simulink model "Main_Sim_Kylle"  (R2018b)
settings: Solver=ode5  StartTime=0.0  StopTime=20000  FixedStep=simParams.sample_time_s  RelTol=1e-3  EnableMultiTasking=on
undefined symbols (not defined in the file or in its folder): DiscIntNeverNeededParam, FSW_Lib, fswParams, MEKF_lib, q_body, r_eci_km, satelliteDynamics_lib, simParams, v_eci_km, w_body_radps
libraries: vrlib x6, aerolibutil x5, CrossProdMatrix_lib x4, sharedutil x4, dspmathops x2, actuators_lib x1, CDH_command_lib x1, Environment_lib x1, MEKF_Conversion_lib x1, sharedtransform x1, actuator_processing_lib x1, allocation_lib x1
(part 1 of 2)
settings Model: Creator=devantormey  LastModifiedBy=kylle
settings OptimizationCC: LifeSpan=inf
settings DebuggingCC: SFUnexpectedBacktrackingDiag=warning  SFNoUnconditionalDefaultTransitionDiag=warning
settings SFSimCC: SimUseLocalCustomCode=off
settings RTWCC: RTWUseLocalCustomCode=off
settings CodeAppCC: StateflowObjectComments=on
settings GRTTargetCC: TargetLangStandard=C89/C90 (ANSI)  GeneratePreprocessorConditionals=Disable all
settings ConfigComp: CovMetricSettings=dw  CovHtmlReporting=on  CovSaveCumulativeToWorkspaceVar=on  CovSaveSingleToWorkspaceVar=on  CovExternalEMLEnable=off

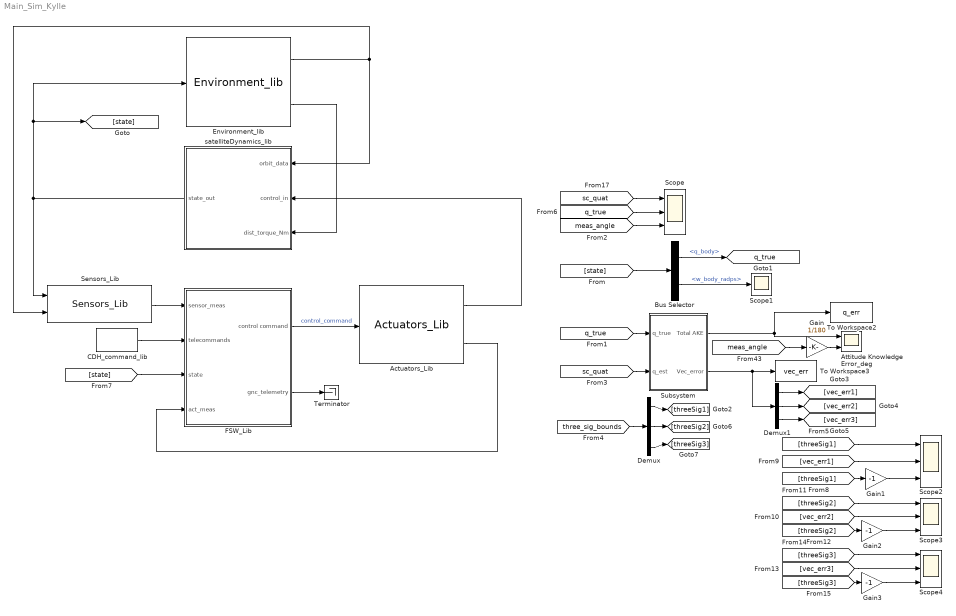
== system Main_Sim_Kylle ==
  Actuators_Lib : actuators_lib/Actuators_Lib  SystemSampleTime=-1
  "Attitude Knowledge Error_deg " : Scope  NumInputPorts=2
  Bus Selector : BusSelector  OutputSignals=q_body,w_body_radps
  CDH_command_lib : CDH_command_lib/CDH_command_lib  SystemSampleTime=-1
  Demux : Demux  Outputs=3
  Demux1 : Demux  Outputs=3
  Environment_lib : Environment_lib/Environment_lib  SystemSampleTime=-1
  FSW_Lib : Subsystem  AncestorBlock=FSW_Lib/FSW_Lib
  Gain : Gain  Gain=1/180
  Gain1 : Gain  Gain=-1
  Gain2 : Gain  Gain=-1
  Gain3 : Gain  Gain=-1
  Scope{,2..4} (4 alike) : Scope  NumInputPorts=3
  Scope1 : Scope
  Sensors_Lib : Sensors_Lib/Sensors_Lib  SystemSampleTime=-1
  Subsystem : Subsystem
  Terminator : Terminator
  To Workspace2 : ToWorkspace  VariableName=q_err  SaveFormat=Timeseries  SampleTime=-1
  To Workspace3 : ToWorkspace  VariableName=vec_err  SaveFormat=Timeseries  SampleTime=-1
  satelliteDynamics_lib : Subsystem  AncestorBlock=satelliteDynamics_lib/satelliteDynamics_lib
  tag scope: q_true=global
  wires:
  FSW_Lib/2(gnc_telemetry) -> Terminator/1
  CDH_command_lib/1 -> FSW_Lib/2(telecommands)
  [state] -> Bus Selector/1
  Bus Selector/2 -> Scope1/1  "<w_body_radps>"
  Bus Selector/1 -> [q_true]  "<q_body>"
  Subsystem/1(Total AKE) -> To Workspace2/1, "Attitude Knowledge Error_deg "/1
  [sc_quat] -> Subsystem/2("q_est ")
  [q_true] -> Subsystem/1("q_true ")
  [q_true] -> Scope/2
  Actuators_Lib/1 -> satelliteDynamics_lib/2(control_in)
  Actuators_Lib/2 -> FSW_Lib/4(act_meas)
  Sensors_Lib/1 -> FSW_Lib/1(sensor_meas)
  FSW_Lib/1(control command) -> Actuators_Lib/1  "control_command"
  [sc_quat] -> Scope/1
  satelliteDynamics_lib/1(state_out) -> Sensors_Lib/1, [state], Environment_lib/1
  Environment_lib/1 -> Sensors_Lib/2, satelliteDynamics_lib/1(orbit_data)
  Environment_lib/2 -> satelliteDynamics_lib/3(dist_torque_Nm)
  [state] -> FSW_Lib/3(state)
  [meas_angle] -> Gain/1
  [meas_angle] -> Scope/3
  [three_sig_bounds] -> Demux/1
  Subsystem/2(Vec_error) -> Demux1/1, To Workspace3/1
  Gain1/1 -> Scope2/3
  Demux/1 -> [threeSig1]
  [threeSig1] -> Scope2/1
  [threeSig1] -> Gain1/1
  Demux1/1 -> [vec_err1]
  Demux1/3 -> [vec_err3]
  Demux1/2 -> [vec_err2]
  [vec_err1] -> Scope2/2
  [vec_err2] -> Scope3/2
  Demux/2 -> [threeSig2]
  Demux/3 -> [threeSig3]
  [threeSig2] -> Scope3/1
  Gain2/1 -> Scope3/3
  [threeSig2] -> Gain2/1
  [threeSig3] -> Scope4/1
  [vec_err3] -> Scope4/2
  [threeSig3] -> Gain3/1
  Gain3/1 -> Scope4/3
  Gain/1 -> "Attitude Knowledge Error_deg "/2

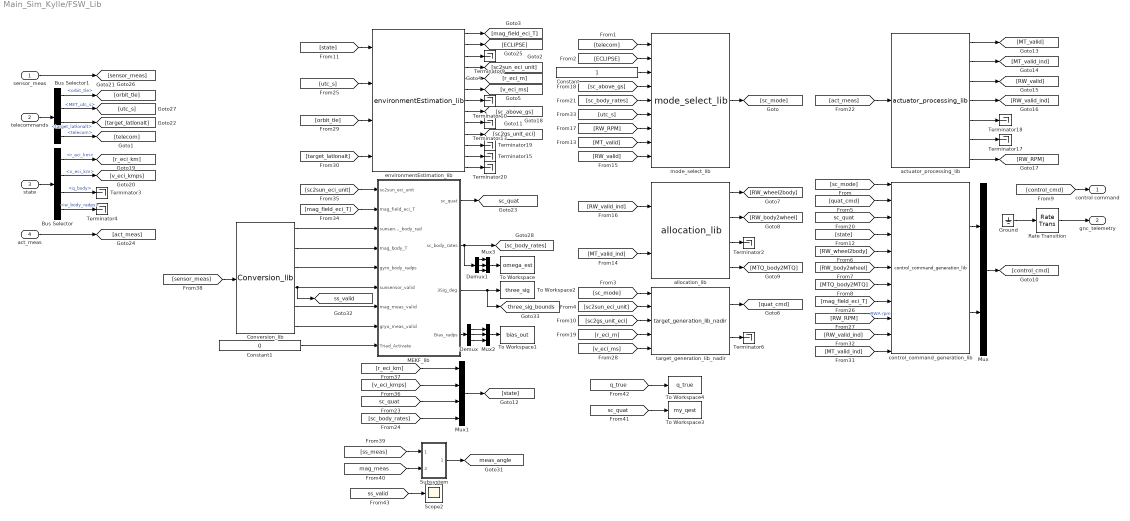
== system Main_Sim_Kylle/FSW_Lib ==
  sensor_meas : Inport
  telecommands : Inport  Port=2
  state : Inport  Port=3
  act_meas : Inport  Port=4
  Bus Selector : BusSelector  OutputSignals=r_eci_km,v_eci_km,q_body,w_body_radps
  Bus Selector1 : BusSelector  OutputSignals=orbit_tle,MET_utc_s,target_latlonalt,telecom
  Constant : Constant
  Constant1 : Constant  Value=0
  Conversion_lib : MEKF_Conversion_lib/Conversion_lib  SystemSampleTime=-1
  Demux : Demux  Outputs=3
  Demux1 : Demux  Outputs=3
  Ground : Ground
  MEKF_lib : Subsystem  AncestorBlock=MEKF_lib/MEKF_lib  TreatAsAtomicUnit=on
      settings: RTWFcnNameOpts=Use subsystem name  RTWFileNameOpts=Use subsystem name
  Mux : Mux  Inputs=[4 5]
  Mux1 : Mux  Inputs=[3 3 4 3]
  Mux2 : Mux  Inputs=3
  Mux3 : Mux  Inputs=3
  Rate Transition : RateTransition  OutPortSampleTime=fswParams.sample_time_s
  Scope2 : Scope
  Subsystem : Subsystem
  Terminator{2..4,6,9..10,13,15,17..20} (12 alike) : Terminator
  To Workspace : ToWorkspace  VariableName=omega_est  SaveFormat=Timeseries  SampleTime=-1
  To Workspace1 : ToWorkspace  VariableName=bias_out  SaveFormat=Timeseries  SampleTime=-1
  To Workspace2 : ToWorkspace  VariableName=three_sig  SaveFormat=Timeseries  SampleTime=-1
  To Workspace3 : ToWorkspace  VariableName=my_qest  SaveFormat=Timeseries  SampleTime=-1
  To Workspace4 : ToWorkspace  VariableName=q_true  SaveFormat=Timeseries  SampleTime=-1
  actuator_processing_lib : actuator_processing_lib/actuator_processing_lib  SystemSampleTime=-1
  allocation_lib : allocation_lib/allocation_lib  SystemSampleTime=-1
  control_command_generation_lib : control_command_generation_lib/control_command_generation_lib  SystemSampleTime=-1
  environmentEstimation_lib : evironmentEstimation_lib/environmentEstimation_lib  SystemSampleTime=-1
  mode_select_lib : mode_select_lib/mode_select_lib  SystemSampleTime=-1
  target_generation_lib_nadir : target_gen_lib_nadir/target_generation_lib_nadir  SystemSampleTime=-1
  control command : Outport
  gnc_telemetry : Outport  Port=2
  tag scope: meas_angle=global, sc_quat=global, ss_valid=global, three_sig_bounds=global
  wires:
  Bus Selector1/4 -> [telecom]  "<telecom>"
  [r_eci_m] -> target_generation_lib_nadir/4
  [utc_s] -> mode_select_lib/6
  [MT_valid_ind] -> control_command_generation_lib/11
  [RW_valid_ind] -> control_command_generation_lib/10
  Rate Transition/1 -> gnc_telemetry/1
  target_generation_lib_nadir/1 -> [quat_cmd]
  [target_latlonalt] -> environmentEstimation_lib/4
  Bus Selector1/3 -> [target_latlonalt]  "<target_latlonalt>"
  Bus Selector1/1 -> [orbit_tle]  "<orbit_tle>"
  [v_eci_ms] -> target_generation_lib_nadir/5
  [RW_RPM] -> control_command_generation_lib/9  "RWA rpm"
  [mag_field_eci_T] -> control_command_generation_lib/8
  Bus Selector1/2 -> [utc_s]  "<MET_utc_s>"
  environmentEstimation_lib/11 -> Terminator19/1
  environmentEstimation_lib/13 -> Terminator20/1
  environmentEstimation_lib/12 -> Terminator15/1
  [act_meas] -> actuator_processing_lib/1
  actuator_processing_lib/7 -> [RW_RPM]
  actuator_processing_lib/6 -> Terminator17/1
  actuator_processing_lib/5 -> Terminator18/1
  actuator_processing_lib/4 -> [RW_valid_ind]
  actuator_processing_lib/3 -> [RW_valid]
  actuator_processing_lib/2 -> [MT_valid_ind]
  actuator_processing_lib/1 -> [MT_valid]
  act_meas/1 -> [act_meas]
  [state] -> control_command_generation_lib/4
  [state] -> environmentEstimation_lib/1
  state/1 -> Bus Selector/1
  [sc2gs_unit_eci] -> target_generation_lib_nadir/3
  [orbit_tle] -> environmentEstimation_lib/3
  [utc_s] -> environmentEstimation_lib/2
  environmentEstimation_lib/10 -> [sc2gs_unit_eci]
  environmentEstimation_lib/9 -> Terminator13/1
  environmentEstimation_lib/8 -> [sc_above_gs]
  environmentEstimation_lib/7 -> Terminator10/1
  environmentEstimation_lib/6 -> [v_eci_ms]
  environmentEstimation_lib/5 -> [r_eci_m]
  environmentEstimation_lib/4 -> [sc2sun_eci_unit]
  environmentEstimation_lib/3 -> Terminator9/1
  environmentEstimation_lib/2 -> [ECLIPSE]
  environmentEstimation_lib/1 -> [mag_field_eci_T]
  Mux/1 -> [control_cmd]
  control_command_generation_lib/1 -> Mux/1
  control_command_generation_lib/2 -> Mux/2
  [MTQ_body2MTQ] -> control_command_generation_lib/7
  [RW_body2wheel] -> control_command_generation_lib/6
  allocation_lib/4 -> [MTQ_body2MTQ]
  allocation_lib/3 -> Terminator2/1
  [RW_wheel2body] -> control_command_generation_lib/5
  allocation_lib/2 -> [RW_body2wheel]
  allocation_lib/1 -> [RW_wheel2body]
  [sc_quat] -> control_command_generation_lib/3
  [MT_valid_ind] -> allocation_lib/2
  [RW_valid_ind] -> allocation_lib/1
  [quat_cmd] -> control_command_generation_lib/2
  target_generation_lib_nadir/2 -> Terminator6/1
  [sc2sun_eci_unit] -> target_generation_lib_nadir/2
  [sc_mode] -> target_generation_lib_nadir/1
  [RW_valid] -> mode_select_lib/9
  [MT_valid] -> mode_select_lib/8
  Constant/1 -> mode_select_lib/3
  [RW_RPM] -> mode_select_lib/7
  [sc_body_rates] -> mode_select_lib/5
  [sc_above_gs] -> mode_select_lib/4
  [ECLIPSE] -> mode_select_lib/2
  [telecom] -> mode_select_lib/1
  [sc_mode] -> control_command_generation_lib/1
  mode_select_lib/1 -> [sc_mode]
  [control_cmd] -> control command/1
  Ground/1 -> Rate Transition/1
  telecommands/1 -> Bus Selector1/1
  [sc_quat] -> Mux1/3
  [sc_body_rates] -> Mux1/4
  Mux1/1 -> [state]
  Conversion_lib/5 -> MEKF_lib/7(mag_meas_valid)
  Conversion_lib/4 -> MEKF_lib/6(sunsensor_valid), [ss_valid]
  Conversion_lib/3 -> MEKF_lib/5(gyro_body_radps)
  Conversion_lib/2 -> MEKF_lib/4(mag_body_T)
  Conversion_lib/1 -> MEKF_lib/3(sunsensor_body_rad)
  [sc2sun_eci_unit] -> MEKF_lib/1(sc2sun_eci_unit)
  [mag_field_eci_T] -> MEKF_lib/2(mag_field_eci_T)
  Bus Selector/1 -> [r_eci_km]  "<r_eci_km>"
  Bus Selector/2 -> [v_eci_kmps]  "<v_eci_km>"
  [r_eci_km] -> Mux1/1
  [v_eci_kmps] -> Mux1/2
  Bus Selector/3 -> Terminator3/1  "<q_body>"
  Bus Selector/4 -> Terminator4/1  "<w_body_radps>"
  sensor_meas/1 -> [sensor_meas]
  [sensor_meas] -> Conversion_lib/1
  MEKF_lib/1(sc_quat) -> [sc_quat]
  MEKF_lib/2(sc_body_rates) -> Demux1/1, [sc_body_rates]
  [ss_meas] -> Subsystem/1(In1)
  [mag_meas] -> Subsystem/2(In2)
  Subsystem/1(Out1) -> [meas_angle]
  [q_true] -> To Workspace4/1
  MEKF_lib/4(Bias_radps) -> Demux/1
  Mux2/1 -> To Workspace1/1
  Demux/1 -> Mux2/1
  Demux/2 -> Mux2/2
  Demux/3 -> Mux2/3
  Demux1/1 -> Mux3/1
  Demux1/2 -> Mux3/2
  Demux1/3 -> Mux3/3
  Mux3/1 -> To Workspace/1
  MEKF_lib/3("3Sig_deg ") -> [three_sig_bounds], To Workspace2/1
  Constant1/1 -> MEKF_lib/9(Triad_Activate)
  Conversion_lib/6 -> MEKF_lib/8(gryo_meas_valid)
  [ss_valid] -> Scope2/1
  [sc_quat] -> To Workspace3/1

== system Main_Sim_Kylle/Subsystem ==
  "q_true " : Inport
  "q_est " : Inport  Port=2
  Acos : Trigonometry  Operator=acos
  Demux3 : Demux
  Gain1 : Gain  Gain=180/pi
  Gain6 : Gain  Gain=180/pi*2
  Mux : Mux  Inputs=3
  Quaternion Conjugate : aerolibutil/Quaternion Conjugate
      settings: SourceProductName=Aerospace Blockset  SourceProductBaseCode=AE
  Quaternion Multiplication : aerolibutil/Quaternion Multiplication
  Total AKE : Outport
  Vec_error : Outport  Port=2
  wires:
  "q_true "/1 -> Quaternion Conjugate/1
  Acos/1 -> Gain6/1
  Mux/1 -> Gain1/1
  Gain6/1 -> Total AKE/1
  Demux3/2 -> Mux/1
  Quaternion Conjugate/1 -> Quaternion Multiplication/1
  Demux3/1 -> Acos/1
  Demux3/3 -> Mux/2
  "q_est "/1 -> Quaternion Multiplication/2
  Demux3/4 -> Mux/3
  Gain1/1 -> Vec_error/1
  Quaternion Multiplication/1 -> Demux3/1

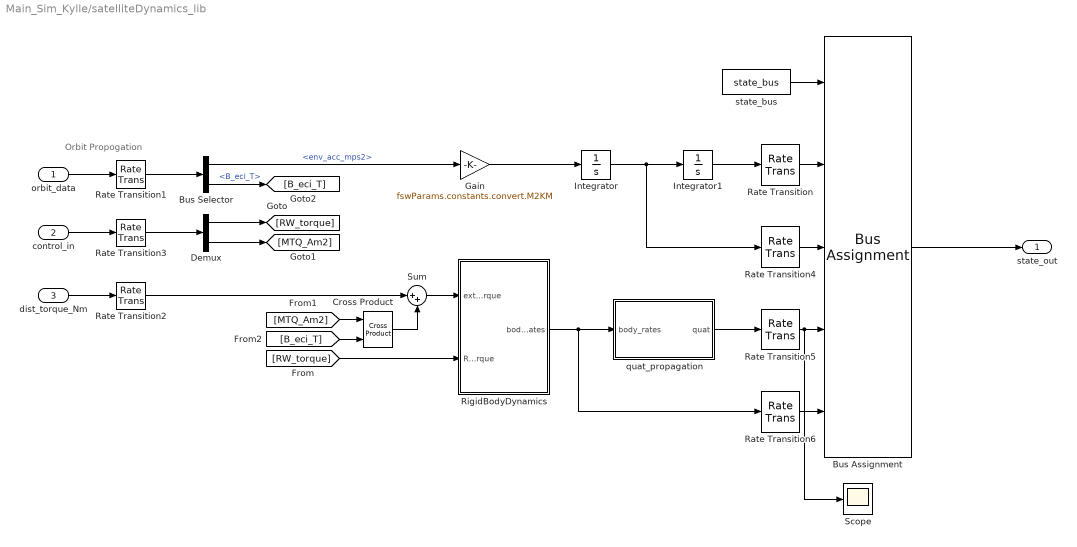
== system Main_Sim_Kylle/satelliteDynamics_lib ==
  note: Orbit Propogation
  orbit_data : Inport
  control_in : Inport  Port=2
  dist_torque_Nm : Inport  Port=3
  Bus Assignment : BusAssignment  AssignedSignals=r_eci_km,v_eci_km,q_body,w_body_radps
  Bus Selector : BusSelector  OutputSignals=env_acc_mps2,B_eci_T
  Cross Product : vrlib/Utilities/Cross Product
      settings: SourceProductBaseCode=VR
  Demux : Demux  Outputs=[3 3]
  Gain : Gain  Gain=fswParams.constants.convert.M2KM
  Integrator : Integrator  InitialCondition=simParams.initialConditions.v0
  Integrator1 : Integrator  InitialCondition=simParams.initialConditions.r0
  Rate Transition : RateTransition  InitialCondition=simParams.initialConditions.r0
  Rate Transition1 : RateTransition  OutPortSampleTime=simParams.sample_time_s
  Rate Transition2 : RateTransition  OutPortSampleTime=simParams.sample_time_s
  Rate Transition3 : RateTransition  OutPortSampleTime=simParams.sample_time_s
  Rate Transition4 : RateTransition  InitialCondition=simParams.initialConditions.v0
  Rate Transition5 : RateTransition  InitialCondition=simParams.initialConditions.q0
  Rate Transition6 : RateTransition  InitialCondition=simParams.initialConditions.w0
  RigidBodyDynamics : Subsystem
  Scope : Scope
  Sum : Sum  Inputs=|++
  quat_propagation : Subsystem
  state_bus : state_bus/state_bus  SystemSampleTime=-1
  state_out : Outport
  wires:
  Rate Transition6/1 -> Bus Assignment/5
  Rate Transition5/1 -> Scope/1, Bus Assignment/4
  Rate Transition4/1 -> Bus Assignment/3
  Rate Transition/1 -> Bus Assignment/2
  state_bus/1 -> Bus Assignment/1
  Sum/1 -> RigidBodyDynamics/1(external_torque)
  [MTQ_Am2] -> Cross Product/1
  [RW_torque] -> RigidBodyDynamics/2(RW_torque)
  Demux/2 -> [MTQ_Am2]
  Demux/1 -> [RW_torque]
  Rate Transition3/1 -> Demux/1
  Rate Transition2/1 -> Sum/1
  RigidBodyDynamics/1(body_rates) -> quat_propagation/1(body_rates), Rate Transition6/1
  quat_propagation/1(quat) -> Rate Transition5/1
  dist_torque_Nm/1 -> Rate Transition2/1
  Bus Assignment/1 -> state_out/1
  Gain/1 -> Integrator/1
  Integrator1/1 -> Rate Transition/1
  Integrator/1 -> Integrator1/1, Rate Transition4/1
  control_in/1 -> Rate Transition3/1
  orbit_data/1 -> Rate Transition1/1
  Bus Selector/1 -> Gain/1  "<env_acc_mps2>"
  Rate Transition1/1 -> Bus Selector/1
  Bus Selector/2 -> [B_eci_T]  "<B_eci_T>"
  [B_eci_T] -> Cross Product/2
  Cross Product/1 -> Sum/2

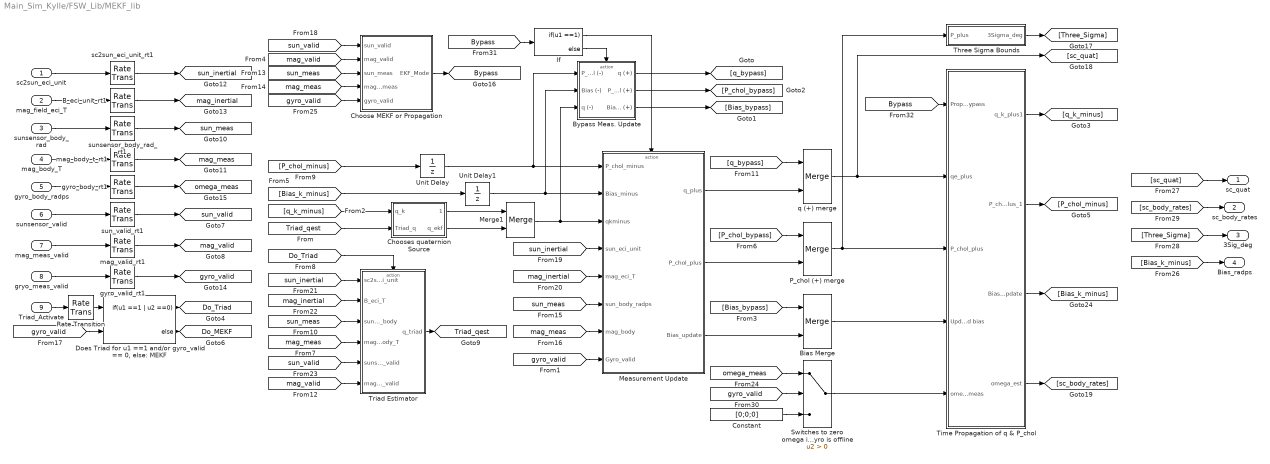
== system Main_Sim_Kylle/FSW_Lib/MEKF_lib ==
  sc2sun_eci_unit : Inport
  mag_field_eci_T : Inport  Port=2
  sunsensor_body_rad : Inport  Port=3
  mag_body_T : Inport  Port=4
  gyro_body_radps : Inport  Port=5
  sunsensor_valid : Inport  Port=6
  mag_meas_valid : Inport  Port=7
  gryo_meas_valid : Inport  Port=8
  Triad_Activate : Inport  Port=9
  B_eci_unit_rt1 : RateTransition  InitialCondition=fswParams.estimation.ic.B_eci_unit_rt  OutPortSampleTime=fswParams.sample_time_s
  Bias Merge : Merge
  Bypass Meas. Update : Subsystem  TreatAsAtomicUnit=on
  Choose MEKF or Propagation : Subsystem
  Chooses quaternion Source : Subsystem
  Constant : Constant  Value=[0;0;0]
  "Does Triad for u1 ==1 and/or gyro_valid == 0, else: MEKF" : If  NumInputs=2  IfExpression=u1 ==1 | u2 ==0
  If : If  IfExpression=u1 ==1
  Measurement Update : Subsystem  TreatAsAtomicUnit=on
  Merge1 : Merge
  P_chol (+) merge : Merge
  Rate Transition : RateTransition  OutPortSampleTime=fswParams.sample_time_s
  "Switches to zero omega if Gyro is offline " : Switch  Criteria=u2 > Threshold
  Three Sigma Bounds : Subsystem
  Time Propagation of q & P_chol : Subsystem
  Triad Estimator : Subsystem  TreatAsAtomicUnit=on
  Unit Delay : UnitDelay  InitialCondition=fswParams.estimation.ic.Pchol_init  SampleTime=fswParams.sample_time_s
  Unit Delay1 : UnitDelay  InitialCondition=fswParams.estimation.ic.Beta_init  SampleTime=fswParams.sample_time_s
  gyro_body_rt1 : RateTransition  InitialCondition=fswParams.estimation.ic.gyro_meas_rt  OutPortSampleTime=fswParams.sample_time_s
  gyro_valid_rt1 : RateTransition  InitialCondition=fswParams.estimation.ic.gyro_valid_rt  OutPortSampleTime=fswParams.sample_time_s
  mag_body_t_rt1 : RateTransition  InitialCondition=fswParams.estimation.ic.mag_body_rt  OutPortSampleTime=fswParams.sample_time_s
  mag_valid_rt1 : RateTransition  InitialCondition=fswParams.estimation.ic.mag_valid_rt  OutPortSampleTime=fswParams.sample_time_s
  q (+) merge : Merge
  sc2sun_eci_unit_rt1 : RateTransition  InitialCondition=fswParams.estimation.ic.sc2sun_eci_unit_rt  OutPortSampleTime=fswParams.sample_time_s
  sun_valid_rt1 : RateTransition  InitialCondition=fswParams.estimation.ic.sun_valid_rt  OutPortSampleTime=fswParams.sample_time_s
  sunsensor_body_rad_rt1 : RateTransition  InitialCondition=fswParams.estimation.ic.sunsensor_body_rad_rt  OutPortSampleTime=fswParams.sample_time_s
  sc_quat : Outport
  sc_body_rates : Outport  Port=2
  "3Sig_deg " : Outport  Port=3
  Bias_radps : Outport  Port=4
  tag scope: Bypass=global, Do_MEKF=global, Do_Triad=global, Triad_qest=global, gyro_valid=global, mag_inertial=global, mag_meas=global, mag_valid=global, omega_meas=global, sun_inertial=global, sun_meas=global, sun_valid=global
  wires:
  [gyro_valid] -> "Switches to zero omega if Gyro is offline "/2
  [Bypass] -> If/1
  [Bypass] -> Time Propagation of q & P_chol/1("Prop_bypass ")
  Bias Merge/1 -> Time Propagation of q & P_chol/4(Updated bias)
  "Switches to zero omega if Gyro is offline "/1 -> Time Propagation of q & P_chol/5(omega_meas)
  [sc_body_rates] -> sc_body_rates/1
  Time Propagation of q & P_chol/4(omega_est) -> [sc_body_rates]
  [Three_Sigma] -> "3Sig_deg "/1
  Three Sigma Bounds/1(3Sigma_deg) -> [Three_Sigma]
  [sc_quat] -> sc_quat/1
  [Bias_k_minus] -> Bias_radps/1
  [gyro_valid] -> Choose MEKF or Propagation/5(gyro_valid)
  [gyro_valid] -> "Does Triad for u1 ==1 and/or gyro_valid == 0, else: MEKF"/2
  [mag_inertial] -> Triad Estimator/2(B_eci_T)
  [mag_valid] -> Triad Estimator/6(magsensor_valid)
  [sun_inertial] -> Triad Estimator/1(sc2sun_eci_unit)
  [mag_meas] -> Triad Estimator/4(mag_meas_body_T)
  [sun_valid] -> Triad Estimator/5(sunsensor_valid)
  [Do_Triad] -> Triad Estimator/Action
  [sun_meas] -> Triad Estimator/3(sun_meas_rad_body)
  [mag_meas] -> Choose MEKF or Propagation/4(mag_meas)
  [sun_meas] -> Choose MEKF or Propagation/3(sun_meas)
  [mag_valid] -> Choose MEKF or Propagation/2(mag_valid)
  [sun_valid] -> Choose MEKF or Propagation/1(sun_valid)
  [gyro_valid] -> Measurement Update/8(Gyro_valid)
  [Triad_qest] -> Chooses quaternion Source/2(Triad_q)
  Chooses quaternion Source/2(q_ekf) -> Merge1/2
  Chooses quaternion Source/1(Triad_qest) -> Merge1/1
  [q_k_minus] -> Chooses quaternion Source/1(q_k)
  Triad Estimator/1(q_triad) -> [Triad_qest]
  [sun_inertial] -> Measurement Update/4(sun_eci_unit)
  [mag_inertial] -> Measurement Update/5("mag_eci_T ")
  [omega_meas] -> "Switches to zero omega if Gyro is offline "/1
  gyro_body_rt1/1 -> [omega_meas]
  gyro_valid_rt1/1 -> [gyro_valid]
  B_eci_unit_rt1/1 -> [mag_inertial]
  sc2sun_eci_unit_rt1/1 -> [sun_inertial]
  Choose MEKF or Propagation/1(EKF_Mode) -> [Bypass]
  Merge1/1 -> Measurement Update/3(qkminus), Bypass Meas. Update/3(q (-))
  Unit Delay1/1 -> Bypass Meas. Update/2(Bias (-)), Measurement Update/2(Bias_minus)
  Unit Delay/1 -> Bypass Meas. Update/1(P_chol (-)), Measurement Update/1(P_chol_minus)
  mag_valid_rt1/1 -> [mag_valid]
  sun_valid_rt1/1 -> [sun_valid]
  [mag_meas] -> Measurement Update/7(mag_body)
  mag_body_t_rt1/1 -> [mag_meas]
  sunsensor_body_rad_rt1/1 -> [sun_meas]
  [sun_meas] -> Measurement Update/6(sun_body_radps)
  gyro_body_radps/1 -> gyro_body_rt1/1
  mag_meas_valid/1 -> mag_valid_rt1/1
  sunsensor_valid/1 -> sun_valid_rt1/1
  "Does Triad for u1 ==1 and/or gyro_valid == 0, else: MEKF"/2 -> [Do_MEKF]
  "Does Triad for u1 ==1 and/or gyro_valid == 0, else: MEKF"/1 -> [Do_Triad]
  Triad_Activate/1 -> Rate Transition/1
  Rate Transition/1 -> "Does Triad for u1 ==1 and/or gyro_valid == 0, else: MEKF"/1
  sunsensor_body_rad/1 -> sunsensor_body_rad_rt1/1
  mag_body_T/1 -> mag_body_t_rt1/1
  mag_field_eci_T/1 -> B_eci_unit_rt1/1
  sc2sun_eci_unit/1 -> sc2sun_eci_unit_rt1/1
  Time Propagation of q & P_chol/1(q_k_plus1) -> [q_k_minus]
  Time Propagation of q & P_chol/2(P_chol_plus_1) -> [P_chol_minus]
  If/1 -> Measurement Update/Action
  If/2 -> Bypass Meas. Update/Action
  [Bias_k_minus] -> Unit Delay1/1
  [P_chol_minus] -> Unit Delay/1
  Measurement Update/1(q_plus) -> q (+) merge/2
  Measurement Update/3(Bias_update) -> Bias Merge/2
  Bypass Meas. Update/1(q (+)) -> [q_bypass]
  [q_bypass] -> q (+) merge/1
  [Bias_bypass] -> Bias Merge/1
  Bypass Meas. Update/2(P_chol (+)) -> [P_chol_bypass]
  Bypass Meas. Update/3(Bias (+)) -> [Bias_bypass]
  gryo_meas_valid/1 -> gyro_valid_rt1/1
  Constant/1 -> "Switches to zero omega if Gyro is offline "/3
  P_chol (+) merge/1 -> Time Propagation of q & P_chol/3(P_chol_plus), Three Sigma Bounds/1(P_plus)
  [P_chol_bypass] -> P_chol (+) merge/1
  Measurement Update/2(P_chol_plus) -> P_chol (+) merge/2
  Time Propagation of q & P_chol/3(Bias_Update) -> [Bias_k_minus]
  q (+) merge/1 -> [sc_quat], Time Propagation of q & P_chol/2(qe_plus)

== system Main_Sim_Kylle/FSW_Lib/Subsystem ==
  In1 : Inport
  In2 : Inport  Port=2
  Acos : Trigonometry  Operator=acos
  Divide : Product  Inputs=*/
  Dot Product : DotProduct  InputSameDT=on  OutDataTypeStr=Inherit: Inherit via internal rule
  Dot Product1 : DotProduct  InputSameDT=on  OutDataTypeStr=Inherit: Inherit via internal rule
  Dot Product2 : DotProduct  InputSameDT=on  OutDataTypeStr=Inherit: Inherit via internal rule
  Gain : Gain  Gain=180/pi
  Multiply : Product
  Sqrt : Sqrt  SaturateOnIntegerOverflow=on
  Sqrt1 : Sqrt  SaturateOnIntegerOverflow=on
  Out1 : Outport
  wires:
  In1/1 -> Dot Product1/2, Dot Product1/1, Dot Product/1
  Divide/1 -> Acos/1
  Dot Product2/1 -> Sqrt1/1
  In2/1 -> Dot Product2/2, Dot Product2/1, Dot Product/2
  Sqrt1/1 -> Multiply/2
  Sqrt/1 -> Multiply/1
  Dot Product/1 -> Divide/1
  Dot Product1/1 -> Sqrt/1
  Multiply/1 -> Divide/2
  Acos/1 -> Gain/1
  Gain/1 -> Out1/1

== system Main_Sim_Kylle/satelliteDynamics_lib/RigidBodyDynamics ==
  external_torque : Inport
  RW_torque : Inport  Port=2
  Discrete-Time Integrator : DiscreteIntegrator  InitialCondition=[0;0;0]  SampleTime=-1  ICPrevOutput=DiscIntNeverNeededParam  ICPrevScaledInput=DiscIntNeverNeededParam
  Integrator : Integrator  InitialCondition=simParams.initialConditions.w0
  dynamics : Subsystem
  body_rates : Outport
  wires:
  dynamics/1(omega_dot) -> Integrator/1
  external_torque/1 -> dynamics/1(external_torque_Nm)
  Integrator/1 -> dynamics/4(omega_radps), body_rates/1
  Discrete-Time Integrator/1 -> dynamics/3(rw_momentum_Nms)
  RW_torque/1 -> Discrete-Time Integrator/1, dynamics/2(rw_torque_Nm)

== system Main_Sim_Kylle/satelliteDynamics_lib/quat_propagation ==
  body_rates : Inport
  Gain1 : Gain  Gain=1/2
  Integrator : Integrator  InitialCondition=simParams.initialConditions.q0
  MATLAB Function : MATLAB Function  TreatAsAtomicUnit=on
  Product : Product  Multiplication=Matrix(*)  RndMeth=Zero
  Quaternion Normalize : sharedutil/Quaternion Normalize  aMode=aMode
      settings: SourceProductName=Aerospace Blockset  SourceProductBaseCode=AE
  quat : Outport
  wires:
  MATLAB Function/1(Omega) -> Gain1/1
  body_rates/1 -> MATLAB Function/1(w)
  Quaternion Normalize/1 -> Product/2, quat/1
  Gain1/1 -> Product/1
  Integrator/1 -> Quaternion Normalize/1
  Product/1 -> Integrator/1

== system Main_Sim_Kylle/FSW_Lib/MEKF_lib/Bypass Meas. Update ==
  P_chol (-) : Inport
  Bias (-) : Inport  Port=2
  q (-) : Inport  Port=3
  Action Port : ActionPort  ActionType=else
  q (+) : Outport
  P_chol (+) : Outport  Port=2
  Bias (+) : Outport  Port=3
  wires:
  P_chol (-)/1 -> P_chol (+)/1
  Bias (-)/1 -> Bias (+)/1
  q (-)/1 -> q (+)/1

== system Main_Sim_Kylle/FSW_Lib/MEKF_lib/Choose MEKF or Propagation ==
  sun_valid : Inport
  mag_valid : Inport  Port=2
  sun_meas : Inport  Port=3
  mag_meas : Inport  Port=4
  gyro_valid : Inport  Port=5
  AND : Logic  Inputs=4  AllPortsSameDT=off  OutDataTypeStr=boolean
  Decides if Angle Between Measurements < 2.5 deg : Subsystem  AncestorBlock=MEKF_lib/MEKF_lib/Triad_alg/Triad/Angle_between_vectors
  EKF_Mode : Outport
  wires:
  gyro_valid/1 -> AND/4
  mag_meas/1 -> Decides if Angle Between Measurements < 2.5 deg/2(mag_meas_T_body)
  sun_meas/1 -> Decides if Angle Between Measurements < 2.5 deg/1(sun_meas_rad_body)
  mag_valid/1 -> AND/2
  sun_valid/1 -> AND/1
  AND/1 -> EKF_Mode/1
  Decides if Angle Between Measurements < 2.5 deg/1(Parallel_Protection) -> AND/3

== system Main_Sim_Kylle/FSW_Lib/MEKF_lib/Chooses quaternion Source ==
  q_k : Inport
  Triad_q : Inport  Port=2
  If Action Subsystem2 : Subsystem  TreatAsAtomicUnit=on
  Unit Delay2 : UnitDelay  InitialCondition=fswParams.estimation.ic.quat_est_init  SampleTime=fswParams.sample_time_s
  Triad_qest : Outport
  q_ekf : Outport  Port=2
  wires:
  Triad_q/1 -> Triad_qest/1
  If Action Subsystem2/1(Out1) -> q_ekf/1
  q_k/1 -> Unit Delay2/1
  [Do_MEKF] -> If Action Subsystem2/Action
  Unit Delay2/1 -> If Action Subsystem2/1(In1)

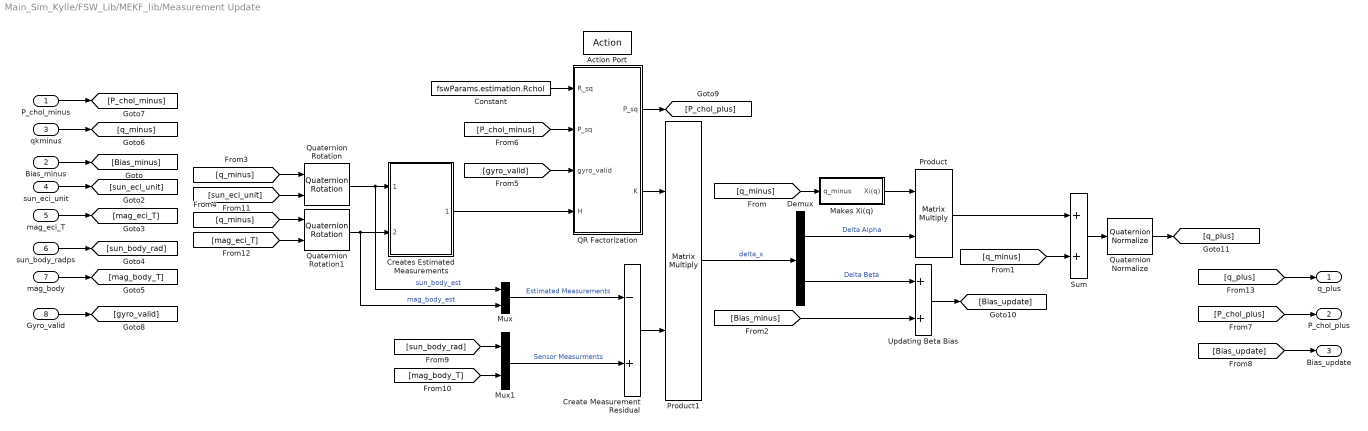
== system Main_Sim_Kylle/FSW_Lib/MEKF_lib/Measurement Update ==
  P_chol_minus : Inport
  Bias_minus : Inport  Port=2
  qkminus : Inport  Port=3
  sun_eci_unit : Inport  Port=4
  "mag_eci_T " : Inport  Port=5
  sun_body_radps : Inport  Port=6
  mag_body : Inport  Port=7
  Gyro_valid : Inport  Port=8
  Action Port : ActionPort  ActionType=then
  Constant : Constant  Value=fswParams.estimation.Rchol  VectorParams1D=off
  Create Measurement Residual : Sum  Inputs=-+
  Creates Estimated Measurements : Subsystem
  Demux : Demux  Outputs=2
  Makes Xi(q) : Subsystem
  Mux : Mux  Inputs=2
  Mux1 : Mux  Inputs=2
  Product : Product  Inputs=**  Multiplication=Matrix(*)
  Product1 : Product  Multiplication=Matrix(*)
  QR Factorization : MATLAB Function  TreatAsAtomicUnit=on
  Quaternion Normalize : sharedutil/Quaternion Normalize  aMode=aMode
      settings: SourceProductName=Aerospace Blockset  SourceProductBaseCode=AE
  Quaternion Rotation : aerolibutil/Quaternion Rotation
  Quaternion Rotation1 : aerolibutil/Quaternion Rotation
  Sum : Sum
  "Updating Beta Bias " : Sum
  q_plus : Outport
  P_chol_plus : Outport  Port=2
  Bias_update : Outport  Port=3
  wires:
  [q_plus] -> q_plus/1
  Quaternion Normalize/1 -> [q_plus]
  [mag_eci_T] -> Quaternion Rotation1/2
  [sun_eci_unit] -> Quaternion Rotation/2
  [mag_body_T] -> Mux1/2
  [sun_body_rad] -> Mux1/1
  Gyro_valid/1 -> [gyro_valid]
  [Bias_update] -> Bias_update/1
  "Updating Beta Bias "/1 -> [Bias_update]
  [P_chol_plus] -> P_chol_plus/1
  QR Factorization/1(P_sq) -> [P_chol_plus]
  [P_chol_minus] -> QR Factorization/2("P_sq ")
  [gyro_valid] -> QR Factorization/3(gyro_valid)
  P_chol_minus/1 -> [P_chol_minus]
  mag_body/1 -> [mag_body_T]
  "mag_eci_T "/1 -> [mag_eci_T]
  sun_eci_unit/1 -> [sun_eci_unit]
  sun_body_radps/1 -> [sun_body_rad]
  [q_minus] -> Quaternion Rotation1/1
  [q_minus] -> Quaternion Rotation/1
  [Bias_minus] -> "Updating Beta Bias "/2
  Bias_minus/1 -> [Bias_minus]
  Constant/1 -> QR Factorization/1(R_sq)
  QR Factorization/2(K) -> Product1/1
  Creates Estimated Measurements/1(H_matrix) -> QR Factorization/4(H)
  [q_minus] -> Makes Xi(q)/1(q_minus)
  qkminus/1 -> [q_minus]
  Quaternion Rotation/1 -> Creates Estimated Measurements/1(sun_body_hat), Mux/1  "sun_body_est"
  Quaternion Rotation1/1 -> Creates Estimated Measurements/2(mag_body_hat), Mux/2  "mag_body_est"
  Create Measurement Residual/1 -> Product1/2
  Makes Xi(q)/1(Xi(q)) -> Product/1
  Demux/1 -> Product/2  "Delta Alpha"
  Product1/1 -> Demux/1  "delta_x"
  Product/1 -> Sum/1
  Sum/1 -> Quaternion Normalize/1
  Mux/1 -> Create Measurement Residual/1  "Estimated Measurements"
  Demux/2 -> "Updating Beta Bias "/1  "Delta Beta"
  Mux1/1 -> Create Measurement Residual/2  "Sensor Measurments"
  [q_minus] -> Sum/2

== system Main_Sim_Kylle/FSW_Lib/MEKF_lib/Three Sigma Bounds ==
  P_plus : Inport
  Abs : Abs
  Demux : Demux  Outputs=2
  Extract Diagonal : S-Function  FunctionName=sdspdiag2  Parameters=mode  SFunctionDeploymentMode=off  EnableBusSupport=off  mask(Extract Diagonal){}
      mask help: Extract the main diagonal of a full matrix.
      mask init:
      | mode = 2;
      | x = [.58 .87 NaN 0.12 0.45 0.45 0.12 0.12 NaN 0.525 0.525 0.475 0.475 0.525 0.525 0.565 0.525 ];
      | y = [ 0.8 0.2 NaN 0.2 0.2 0.8 0.8 0.2 NaN 0.435 0.475 0.475 0.525 0.525 0.565 0.5 0.435 ];
      mask Help: eval('blocksethelp');
      mask Display:
      | plot(x,y);
      | port_label('input',1,'A');
      | port_label('output',1,'D');
  Multiply : Gain  Gain=3*180/pi
  Terminator : Terminator
  3Sigma_deg : Outport
  wires:
  Demux/2 -> Terminator/1
  Demux/1 -> Abs/1
  Extract Diagonal/1 -> Demux/1
  Abs/1 -> Multiply/1
  P_plus/1 -> Extract Diagonal/1
  Multiply/1 -> 3Sigma_deg/1

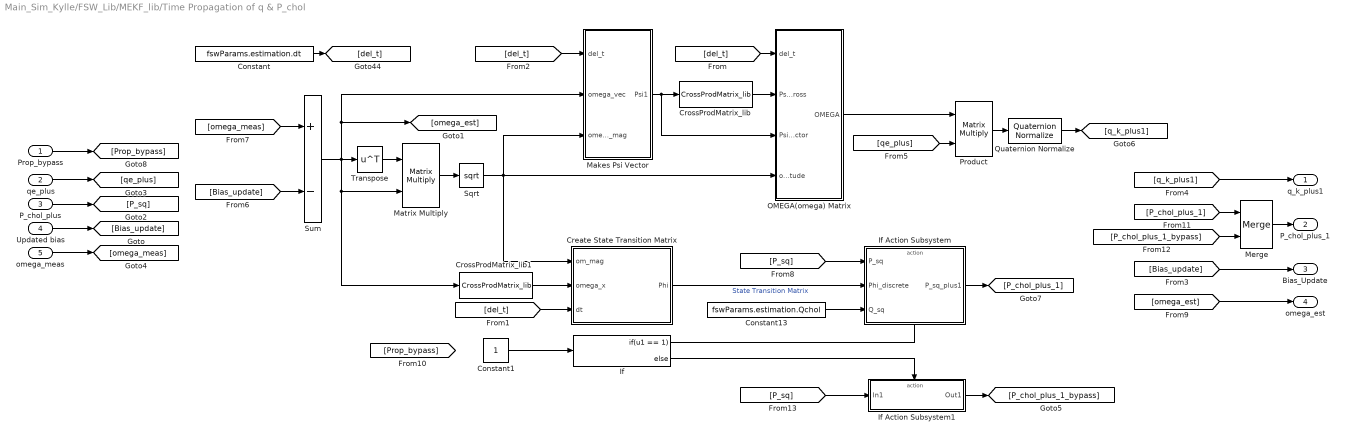
== system Main_Sim_Kylle/FSW_Lib/MEKF_lib/Time Propagation of q & P_chol ==
  "Prop_bypass " : Inport
  qe_plus : Inport  Port=2
  P_chol_plus : Inport  Port=3
  Updated bias : Inport  Port=4
  omega_meas : Inport  Port=5
  Constant : Constant  Value=fswParams.estimation.dt
  Constant1 : Constant
  Constant13 : Constant  Value=fswParams.estimation.Qchol  VectorParams1D=off
  Create State Transition Matrix : MATLAB Function  TreatAsAtomicUnit=on
  CrossProdMatrix_lib : CrossProdMatrix_lib/CrossProdMatrix_lib  SystemSampleTime=-1
  CrossProdMatrix_lib1 : CrossProdMatrix_lib/CrossProdMatrix_lib  SystemSampleTime=-1
  If : If  IfExpression=u1 == 1
  If Action Subsystem : Subsystem  TreatAsAtomicUnit=on
  If Action Subsystem1 : Subsystem  TreatAsAtomicUnit=on
  Makes Psi Vector : Subsystem
  Matrix Multiply : Product  Multiplication=Matrix(*)
  Merge : Merge
  OMEGA(omega) Matrix : Subsystem
  Product : Product  Multiplication=Matrix(*)
  Quaternion Normalize : sharedutil/Quaternion Normalize  aMode=aMode
      settings: SourceProductName=Aerospace Blockset  SourceProductBaseCode=AE
  Sqrt : Sqrt  SaturateOnIntegerOverflow=on
  Sum : Sum  Inputs=+-
  Transpose : Math  Operator=transpose  SaturateOnIntegerOverflow=on
  q_k_plus1 : Outport
  P_chol_plus_1 : Outport  Port=2
  Bias_Update : Outport  Port=3
  omega_est : Outport  Port=4
  wires:
  [P_sq] -> If Action Subsystem1/1(In1)
  "Prop_bypass "/1 -> [Prop_bypass]
  [P_chol_plus_1] -> Merge/1
  Merge/1 -> P_chol_plus_1/1
  [P_chol_plus_1_bypass] -> Merge/2
  If Action Subsystem1/1(Out1) -> [P_chol_plus_1_bypass]
  If/2 -> If Action Subsystem1/Action
  If/1 -> If Action Subsystem/Action
  If Action Subsystem/1(P_sq_plus1) -> [P_chol_plus_1]
  [q_k_plus1] -> q_k_plus1/1
  Quaternion Normalize/1 -> [q_k_plus1]
  [P_sq] -> If Action Subsystem/1("P_sq ")
  [omega_meas] -> Sum/1
  [Bias_update] -> Sum/2
  omega_meas/1 -> [omega_meas]
  P_chol_plus/1 -> [P_sq]
  Updated bias/1 -> [Bias_update]
  [qe_plus] -> Product/2
  qe_plus/1 -> [qe_plus]
  [omega_est] -> omega_est/1
  [Bias_update] -> Bias_Update/1
  Constant13/1 -> If Action Subsystem/3(Q_sq)
  Create State Transition Matrix/1(Phi) -> If Action Subsystem/2(Phi_discrete)  "State Transition Matrix"
  OMEGA(omega) Matrix/1(OMEGA) -> Product/1
  CrossProdMatrix_lib/1 -> OMEGA(omega) Matrix/2(Psi_cross)
  Makes Psi Vector/1(Psi1) -> OMEGA(omega) Matrix/3(Psi_vector), CrossProdMatrix_lib/1
  [del_t] -> OMEGA(omega) Matrix/1(del_t)
  CrossProdMatrix_lib1/1 -> Create State Transition Matrix/2(omega_x)
  Sqrt/1 -> Create State Transition Matrix/1(om_mag), Makes Psi Vector/3(omega_mag), OMEGA(omega) Matrix/4(omega_magnitude)
  Transpose/1 -> Matrix Multiply/1
  Matrix Multiply/1 -> Sqrt/1
  Constant/1 -> [del_t]
  Sum/1 -> Makes Psi Vector/2(omega_vec), [omega_est], CrossProdMatrix_lib1/1, Matrix Multiply/2, Transpose/1
  [del_t] -> Makes Psi Vector/1(del_t)
  [del_t] -> Create State Transition Matrix/3(dt)
  Product/1 -> Quaternion Normalize/1
  Constant1/1 -> If/1

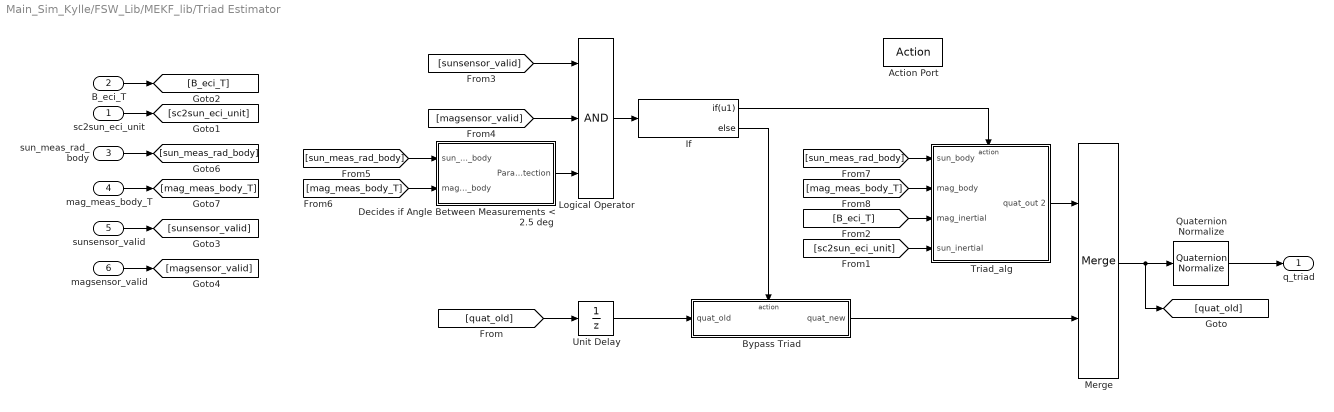
== system Main_Sim_Kylle/FSW_Lib/MEKF_lib/Triad Estimator ==
  sc2sun_eci_unit : Inport
  B_eci_T : Inport  Port=2
  sun_meas_rad_body : Inport  Port=3
  mag_meas_body_T : Inport  Port=4
  sunsensor_valid : Inport  Port=5
  magsensor_valid : Inport  Port=6
  Action Port : ActionPort  ActionType=then
  Bypass Triad : Subsystem  TreatAsAtomicUnit=on
  Decides if Angle Between Measurements < 2.5 deg : Subsystem
  If : If  IfExpression=u1
  Logical Operator : Logic  Inputs=3  AllPortsSameDT=off  OutDataTypeStr=boolean
  Merge : Merge
  Quaternion Normalize : sharedutil/Quaternion Normalize  aMode=aMode
      settings: SourceProductName=Aerospace Blockset  SourceProductBaseCode=AE
  Triad_alg : Subsystem  TreatAsAtomicUnit=on
  Unit Delay : UnitDelay  InitialCondition=fswParams.estimation.ic.quat_est_init  SampleTime=fswParams.sample_time_s
  q_triad : Outport
  wires:
  Quaternion Normalize/1 -> q_triad/1
  [B_eci_T] -> Triad_alg/3("mag_inertial ")
  [sc2sun_eci_unit] -> Triad_alg/4(sun_inertial)
  B_eci_T/1 -> [B_eci_T]
  sc2sun_eci_unit/1 -> [sc2sun_eci_unit]
  [mag_meas_body_T] -> Decides if Angle Between Measurements < 2.5 deg/2(mag_meas_T_body)
  mag_meas_body_T/1 -> [mag_meas_body_T]
  [sun_meas_rad_body] -> Decides if Angle Between Measurements < 2.5 deg/1(sun_meas_rad_body)
  sun_meas_rad_body/1 -> [sun_meas_rad_body]
  [magsensor_valid] -> Logical Operator/2
  magsensor_valid/1 -> [magsensor_valid]
  [sunsensor_valid] -> Logical Operator/1
  sunsensor_valid/1 -> [sunsensor_valid]
  [mag_meas_body_T] -> Triad_alg/2(mag_body)
  [sun_meas_rad_body] -> Triad_alg/1(sun_body)
  Decides if Angle Between Measurements < 2.5 deg/1(Parallel_Protection) -> Logical Operator/3
  Unit Delay/1 -> Bypass Triad/1(quat_old)
  [quat_old] -> Unit Delay/1
  Logical Operator/1 -> If/1
  Bypass Triad/1(quat_new) -> Merge/2
  Triad_alg/1(quat_out 2) -> Merge/1
  If/2 -> Bypass Triad/Action
  If/1 -> Triad_alg/Action
  Merge/1 -> [quat_old], Quaternion Normalize/1

== system Main_Sim_Kylle/satelliteDynamics_lib/RigidBodyDynamics/dynamics ==
  note: Euler's equation: J dw/dt = T_{ext} + T_{rw} - w x ( Jw + h_w )
      |
      | RW being momentum exchange devices do NOT create
      | an external torque on the s/c
  external_torque_Nm : Inport
  rw_torque_Nm : Inport  Port=2
  rw_momentum_Nms : Inport  Port=3
  omega_radps : Inport  Port=4
  Add : Sum  Inputs=|++
  Cross Product : vrlib/Utilities/Cross Product
      settings: SourceProductBaseCode=VR
  Invert  3x3 Matrix : aerolibutil/Invert  3x3 Matrix
  Product : Product  Multiplication=Matrix(*)  RndMeth=Zero
  Product1 : Product  Multiplication=Matrix(*)  RndMeth=Zero
  Sum : Sum  Inputs=+-+
  inertia_tensor1 : Constant  Value=simParams.scParams.J
  inertia_tensor2 : Constant  Value=simParams.scParams.J
  omega_dot : Outport
  wires:
  rw_momentum_Nms/1 -> Add/2
  external_torque_Nm/1 -> Sum/1
  omega_radps/1 -> Product/2, Cross Product/1
  inertia_tensor2/1 -> Product/1
  Sum/1 -> Product1/2
  Product1/1 -> omega_dot/1
  Invert  3x3 Matrix/1 -> Product1/1
  inertia_tensor1/1 -> Invert  3x3 Matrix/1
  Cross Product/1 -> Sum/2
  Product/1 -> Add/1
  Add/1 -> Cross Product/2
  rw_torque_Nm/1 -> Sum/3

== system Main_Sim_Kylle/FSW_Lib/MEKF_lib/Choose MEKF or Propagation/Decides if Angle Between Measurements < 2.5 deg ==
  sun_meas_rad_body : Inport
  mag_meas_T_body : Inport  Port=2
  Divide : Product  Inputs=*/
  Dot Product : DotProduct  InputSameDT=on  OutDataTypeStr=Inherit: Inherit via internal rule
  Dot Product1 : DotProduct  InputSameDT=on  OutDataTypeStr=Inherit: Inherit via internal rule
  Dot Product2 : DotProduct  InputSameDT=on  OutDataTypeStr=Inherit: Inherit via internal rule
  MATLAB Function : MATLAB Function  TreatAsAtomicUnit=on
  Multiply : Product
  Sqrt : Sqrt  SaturateOnIntegerOverflow=on
  Sqrt1 : Sqrt  SaturateOnIntegerOverflow=on
  Parallel_Protection : Outport
  wires:
  MATLAB Function/1(y) -> Parallel_Protection/1
  Divide/1 -> MATLAB Function/1(u)
  Multiply/1 -> Divide/2
  Dot Product2/1 -> Sqrt1/1
  Dot Product/1 -> Divide/1
  Sqrt/1 -> Multiply/1
  Sqrt1/1 -> Multiply/2
  sun_meas_rad_body/1 -> Dot Product/1, Dot Product1/2, Dot Product1/1
  mag_meas_T_body/1 -> Dot Product/2, Dot Product2/1, Dot Product2/2
  Dot Product1/1 -> Sqrt/1

== system Main_Sim_Kylle/FSW_Lib/MEKF_lib/Chooses quaternion Source/If Action Subsystem2 ==
  In1 : Inport
  Action Port : ActionPort  ActionType=else
  Out1 : Outport
  wires:
  In1/1 -> Out1/1

== system Main_Sim_Kylle/FSW_Lib/MEKF_lib/Measurement Update/Creates Estimated Measurements ==
  sun_body_hat : Inport
  mag_body_hat : Inport  Port=2
  Constant1 : Constant  Value=zeros(3,3)  VectorParams1D=off
  Constant2 : Constant  Value=zeros(3,3)  VectorParams1D=off
  CrossProdMatrix_lib : CrossProdMatrix_lib/CrossProdMatrix_lib  SystemSampleTime=-1
  CrossProdMatrix_lib1 : CrossProdMatrix_lib/CrossProdMatrix_lib  SystemSampleTime=-1
  Horizontal Matrix Concatenate : Concatenate  Mode=Multidimensional array
  Horizontal Matrix Concatenate1 : Concatenate  Mode=Multidimensional array
  Vertical Matrix Concatenate : Concatenate  Mode=Multidimensional array  ConcatenateDimension=2
  H_matrix : Outport
  wires:
  Constant1/1 -> Horizontal Matrix Concatenate1/2
  Constant2/1 -> Horizontal Matrix Concatenate1/1
  CrossProdMatrix_lib1/1 -> Horizontal Matrix Concatenate/2
  Horizontal Matrix Concatenate/1 -> Vertical Matrix Concatenate/1
  Horizontal Matrix Concatenate1/1 -> Vertical Matrix Concatenate/2
  sun_body_hat/1 -> CrossProdMatrix_lib/1
  CrossProdMatrix_lib/1 -> Horizontal Matrix Concatenate/1
  mag_body_hat/1 -> CrossProdMatrix_lib1/1
  Vertical Matrix Concatenate/1 -> H_matrix/1

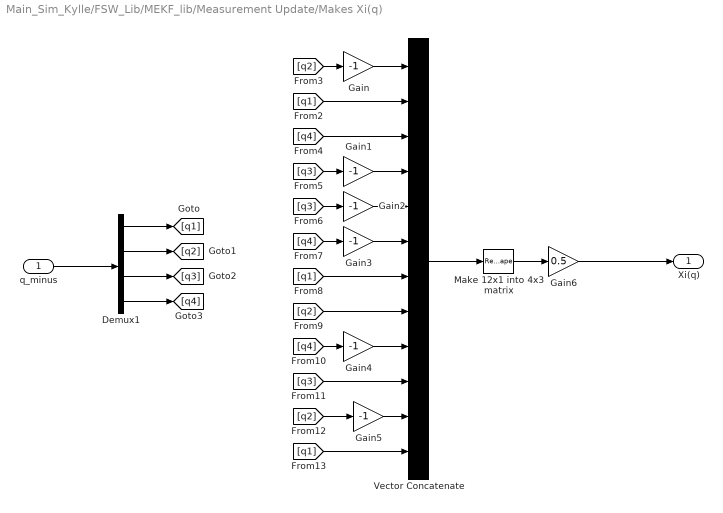
== system Main_Sim_Kylle/FSW_Lib/MEKF_lib/Measurement Update/Makes Xi(q) ==
  q_minus : Inport
  Demux1 : Demux
  Gain{,1..5} (6 alike) : Gain  Gain=-1
  Gain6 : Gain  Gain=0.5
  Make 12x1 into 4x3 matrix : Reshape  OutputDimensionality=Customize  OutputDimensions=[4,3]
  Vector Concatenate : Concatenate  NumInputs=12
  Xi(q) : Outport
  wires:
  Vector Concatenate/1 -> Make 12x1 into 4x3 matrix/1
  [q3] -> Gain2/1
  Gain3/1 -> Vector Concatenate/6
  [q1] -> Vector Concatenate/2
  Make 12x1 into 4x3 matrix/1 -> Gain6/1
  [q3] -> Gain1/1
  [q4] -> Gain3/1
  [q2] -> Gain/1
  [q3] -> Vector Concatenate/10
  Gain2/1 -> Vector Concatenate/5
  Gain1/1 -> Vector Concatenate/4
  Demux1/2 -> [q2]
  [q2] -> Vector Concatenate/8
  Demux1/1 -> [q1]
  Gain4/1 -> Vector Concatenate/9
  Demux1/3 -> [q3]
  [q4] -> Vector Concatenate/3
  [q1] -> Vector Concatenate/12
  Gain/1 -> Vector Concatenate/1
  [q2] -> Gain5/1
  [q4] -> Gain4/1
  Gain5/1 -> Vector Concatenate/11
  [q1] -> Vector Concatenate/7
  Demux1/4 -> [q4]
  q_minus/1 -> Demux1/1
  Gain6/1 -> Xi(q)/1

== system Main_Sim_Kylle/FSW_Lib/MEKF_lib/Time Propagation of q & P_chol/If Action Subsystem ==
  "P_sq " : Inport
  Phi_discrete : Inport  Port=2
  Q_sq : Inport  Port=3
  Action Port : ActionPort  ActionType=then
  Time Propagation of P_chol via QR Decomposition : MATLAB Function  TreatAsAtomicUnit=on
  P_sq_plus1 : Outport
  wires:
  Time Propagation of P_chol via QR Decomposition/1(P_sq) -> P_sq_plus1/1
  Q_sq/1 -> Time Propagation of P_chol via QR Decomposition/3(Q_sq)
  Phi_discrete/1 -> Time Propagation of P_chol via QR Decomposition/2(Phi_discrete)
  "P_sq "/1 -> Time Propagation of P_chol via QR Decomposition/1("P_sq ")

== system Main_Sim_Kylle/FSW_Lib/MEKF_lib/Time Propagation of q & P_chol/If Action Subsystem1 ==
  In1 : Inport
  Action Port : ActionPort  ActionType=else
  Out1 : Outport
  wires:
  In1/1 -> Out1/1

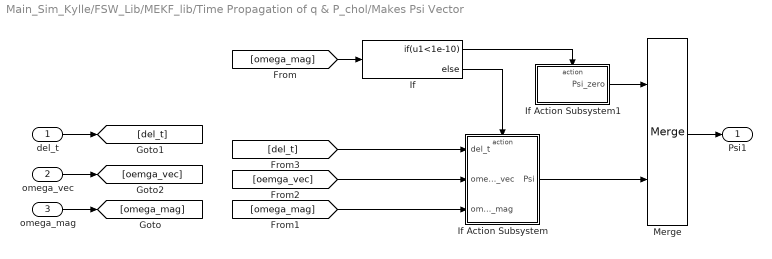
== system Main_Sim_Kylle/FSW_Lib/MEKF_lib/Time Propagation of q & P_chol/Makes Psi Vector ==
  del_t : Inport
  omega_vec : Inport  Port=2
  omega_mag : Inport  Port=3
  If : If  IfExpression=u1<1e-10
  If Action Subsystem : Subsystem  TreatAsAtomicUnit=on
  If Action Subsystem1 : Subsystem  TreatAsAtomicUnit=on
  Merge : Merge
  Psi1 : Outport
  wires:
  [del_t] -> If Action Subsystem/1(del_t)
  [oemga_vec] -> If Action Subsystem/2(omega_vec)
  del_t/1 -> [del_t]
  omega_vec/1 -> [oemga_vec]
  [omega_mag] -> If/1
  [omega_mag] -> If Action Subsystem/3(omega_mag)
  omega_mag/1 -> [omega_mag]
  Merge/1 -> Psi1/1
  If Action Subsystem1/1(Psi_zero) -> Merge/1
  If/1 -> If Action Subsystem1/Action
  If Action Subsystem/1(Psi) -> Merge/2
  If/2 -> If Action Subsystem/Action

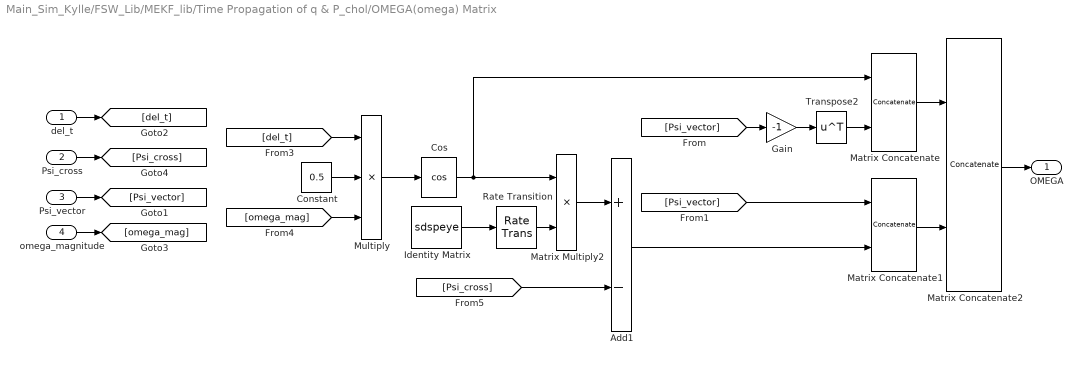
== system Main_Sim_Kylle/FSW_Lib/MEKF_lib/Time Propagation of q & P_chol/OMEGA(omega) Matrix ==
  del_t : Inport
  Psi_cross : Inport  Port=2
  Psi_vector : Inport  Port=3
  omega_magnitude : Inport  Port=4
  Add1 : Sum  Inputs=+-
  Constant : Constant  Value=0.5
  Cos : Trigonometry  Operator=cos
  Gain : Gain  Gain=-1
  Identity Matrix : S-Function  FunctionName=sdspeye  Parameters=Inherit,N,Ts,isCustomFloat,fxpIsSigned,dTypeID,fxpWordLength,fxpFracLength,1  SFunctionDeploymentMode=off  EnableBusSupport=off  mask(Identity Matrix){Inherit=off, N=3, Ts=1, additionalParams=off, allowOverrides=on, dataType=double, isSigned=on, wordLen=16, udDataType=sfix(16), fracBitsMode=Best precision, numFracBits=15, OutDataTypeStr=double, LastOutDataTypeStr=double}
      mask prompts: Inherit "Inherit output port attributes from input port"; N "Matrix size:"; Ts "Sample time:"; additionalParams "------- Show additional parameters --------"; allowOverrides "Allow overrides by DSP Fixed-Point Attributes blocks"; dataType "Output data type:"; isSigned "Signed"; wordLen "Word length:"; udDataType "User-defined data type (e.g. sfix(16), float('single')):"; fracBitsMode "Set fraction length in output to:"; numFracBits "Fraction length:"; OutDataTypeStr "Output data type:"; LastOutDataTypeStr "Last output data type:"
      mask help: Output an identity matrix. If the matrix size entered is a scalar, then the output will be a square (symmetric) identity matrix with the number of rows and columns both equal to the specified value. If the matrix size entered is a two-element vector [M N], then the output will be an asymmetric matrix with the number of rows equal to M, the number of columns equal to N, ones down the diagonal, and zeros elsewhere. This matches the syntax of the MATLAB function eye(N) and eye(M,N), respectively.
      mask init:
      | isCustomFloat =  0; % nice default
      | fxpIsSigned   =  1; % nice default
      | fxpWordLength =  8; % nice default
      | fxpFracLength =  0; % nice default
      | if Inherit
      |     dTypeID   = -3; % SAME_AS_INPUT
      | else
      |     dtRows            = dspblkGetDiscreteImpulseDTRowInfo();
      |     [dtInfo, dTypeID] = dspblkUDTMapperOutDType(gcbh, dtRows{1}, 'dataType', 1.0);
      |     isCustomFloat     = dtInfo.DataTypeIsCustomFloat;
      |     if ~isCustomFloat
      |         fxpIsSigned   = dtInfo.DataTypeIsSigned;
      |         fxpWordLength = dtInfo.DataTypeWordLength;
      |         fxpFracLength = dtInfo.DataTypeFracOrMantBits;
      |     end
      | end
      mask Help: eval('blocksethelp');
      mask Callback Inherit: dspblkeye
      mask TypeOptions dataType: double | single | int8 | uint8 | int16 | uint16 | int32 | uint32 | boolean | Fixed-point | User-defined | Inherit via back propagation
      mask TypeOptions fracBitsMode: Best precision | User-defined
      mask Display:
      | if Inherit
      |     disp('eye( )');
      | else
      |     disp(['eye(' , num2str(get_param(gcbh, 'N')), ')']);
      | end
  Matrix Concatenate : Concatenate  Mode=Multidimensional array  ConcatenateDimension=2
  Matrix Concatenate1 : Concatenate  Mode=Multidimensional array  ConcatenateDimension=2
  Matrix Concatenate2 : Concatenate  Mode=Multidimensional array
  Matrix Multiply2 : Product
  Multiply : Product  Inputs=3
  Rate Transition : RateTransition  InitialCondition=eye(3)  OutPortSampleTime=fswParams.sample_time_s
  Transpose2 : Math  Operator=transpose  SaturateOnIntegerOverflow=on
  OMEGA : Outport
  wires:
  Rate Transition/1 -> Matrix Multiply2/2
  Identity Matrix/1 -> Rate Transition/1
  [Psi_cross] -> Add1/2
  Psi_cross/1 -> [Psi_cross]
  [omega_mag] -> Multiply/3
  omega_magnitude/1 -> [omega_mag]
  [del_t] -> Multiply/1
  del_t/1 -> [del_t]
  [Psi_vector] -> Matrix Concatenate1/1
  [Psi_vector] -> Gain/1
  Psi_vector/1 -> [Psi_vector]
  Gain/1 -> Transpose2/1
  Constant/1 -> Multiply/2
  Transpose2/1 -> Matrix Concatenate/2
  Cos/1 -> Matrix Concatenate/1, Matrix Multiply2/1
  Matrix Concatenate/1 -> Matrix Concatenate2/1
  Matrix Concatenate1/1 -> Matrix Concatenate2/2
  Add1/1 -> Matrix Concatenate1/2
  Matrix Multiply2/1 -> Add1/1
  Multiply/1 -> Cos/1
  Matrix Concatenate2/1 -> OMEGA/1

== system Main_Sim_Kylle/FSW_Lib/MEKF_lib/Triad Estimator/Bypass Triad ==
  quat_old : Inport
  Action Port : ActionPort  ActionType=else
  quat_new : Outport
  wires:
  quat_old/1 -> quat_new/1

== system Main_Sim_Kylle/FSW_Lib/MEKF_lib/Triad Estimator/Decides if Angle Between Measurements < 2.5 deg ==
  sun_meas_rad_body : Inport
  mag_meas_T_body : Inport  Port=2
  Divide : Product  Inputs=*/
  Dot Product : DotProduct  InputSameDT=on  OutDataTypeStr=Inherit: Inherit via internal rule
  Dot Product1 : DotProduct  InputSameDT=on  OutDataTypeStr=Inherit: Inherit via internal rule
  Dot Product2 : DotProduct  InputSameDT=on  OutDataTypeStr=Inherit: Inherit via internal rule
  MATLAB Function : MATLAB Function  TreatAsAtomicUnit=on
  Multiply : Product
  Sqrt : Sqrt  SaturateOnIntegerOverflow=on
  Sqrt1 : Sqrt  SaturateOnIntegerOverflow=on
  Parallel_Protection : Outport
  wires:
  MATLAB Function/1(y) -> Parallel_Protection/1
  Divide/1 -> MATLAB Function/1(u)
  Multiply/1 -> Divide/2
  Dot Product2/1 -> Sqrt1/1
  Dot Product/1 -> Divide/1
  Sqrt/1 -> Multiply/1
  Sqrt1/1 -> Multiply/2
  sun_meas_rad_body/1 -> Dot Product/1, Dot Product1/2, Dot Product1/1
  mag_meas_T_body/1 -> Dot Product/2, Dot Product2/1, Dot Product2/2
  Dot Product1/1 -> Sqrt/1

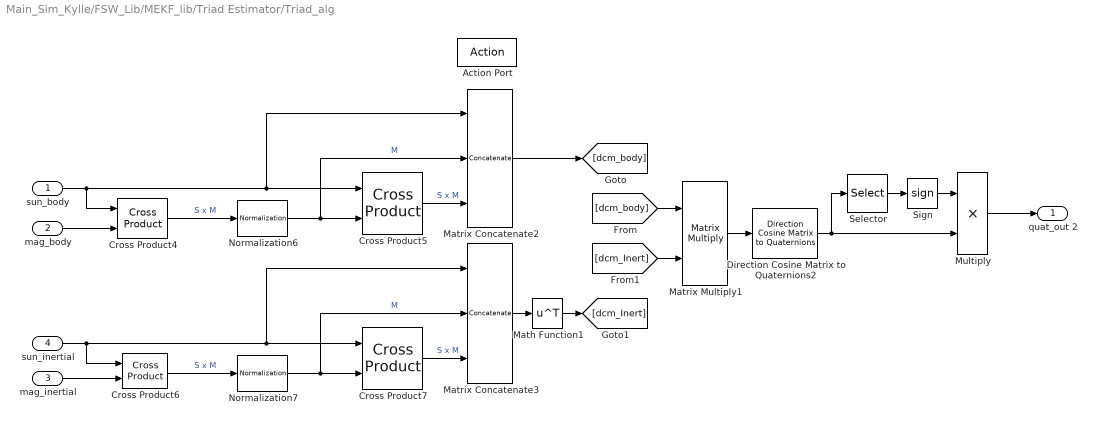
== system Main_Sim_Kylle/FSW_Lib/MEKF_lib/Triad Estimator/Triad_alg ==
  sun_body : Inport
  mag_body : Inport  Port=2
  "mag_inertial " : Inport  Port=3
  sun_inertial : Inport  Port=4
  Action Port : ActionPort  ActionType=then
  Cross Product{4..7} (4 alike) : vrlib/Utilities/Cross Product
      settings: SourceProductBaseCode=VR
  Direction Cosine Matrix to Quaternions2 : sharedtransform/Direction Cosine Matrix  to Quaternions  aMode=0  action=None  tolerance=eps(2)
      settings: SourceProductName=Aerospace Blockset  SourceProductBaseCode=AE
  Math Function1 : Math  Operator=transpose  SaturateOnIntegerOverflow=on
  Matrix Concatenate2 : Concatenate  NumInputs=3  Mode=Multidimensional array  ConcatenateDimension=2
  Matrix Concatenate3 : Concatenate  NumInputs=3  Mode=Multidimensional array  ConcatenateDimension=2
  Matrix Multiply1 : Product  Multiplication=Matrix(*)
  Multiply : Product
  Normalization6 : dspmathops/Normalization  NormType=2-norm  Bias=1e-10  NormOver=Each column  Dimension=1  roundingMode=Floor  overflowMode=off  accumDataTypeStr=Inherit: Same as product output  accumLastDataTypeStr=Inherit: Same as product output  outputDataTypeStr=Inherit: Same as product output  outputMin=[]  outputMax=[]  outputLastDataTypeStr=Inherit: Same as product output
      settings: SourceProductName=DSP System Toolbox
  Normalization7 : dspmathops/Normalization  NormType=2-norm  Bias=1e-10  NormOver=Each column  Dimension=1  roundingMode=Floor  overflowMode=off  accumDataTypeStr=Inherit: Same as product output  accumLastDataTypeStr=Inherit: Same as product output  outputDataTypeStr=Inherit: Same as product output  outputMin=[]  outputMax=[]  outputLastDataTypeStr=Inherit: Same as product output
      settings: SourceProductName=DSP System Toolbox
  Selector : Selector  InputPortWidth=4  IndexOptions=Index vector (dialog)  Indices=[1]  OutputSizes=1
  Sign : Signum
  quat_out 2 : Outport
  wires:
  Multiply/1 -> quat_out 2/1
  Selector/1 -> Sign/1
  Sign/1 -> Multiply/1
  Direction Cosine Matrix to Quaternions2/1 -> Selector/1, Multiply/2
  [dcm_Inert] -> Matrix Multiply1/2
  [dcm_body] -> Matrix Multiply1/1
  Math Function1/1 -> [dcm_Inert]
  Matrix Concatenate2/1 -> [dcm_body]
  Matrix Multiply1/1 -> Direction Cosine Matrix to Quaternions2/1
  Matrix Concatenate3/1 -> Math Function1/1
  "mag_inertial "/1 -> Cross Product6/2
  Cross Product6/1 -> Normalization7/1  "S x M"
  Normalization7/1 -> Cross Product7/2, Matrix Concatenate3/2  "M"
  Cross Product7/1 -> Matrix Concatenate3/3  "S x M"
  sun_inertial/1 -> Cross Product7/1, Matrix Concatenate3/1, Cross Product6/1
  Cross Product5/1 -> Matrix Concatenate2/3  "S x M"
  Normalization6/1 -> Cross Product5/2, Matrix Concatenate2/2  "M"
  Cross Product4/1 -> Normalization6/1  "S x M"
  mag_body/1 -> Cross Product4/2
  sun_body/1 -> Cross Product4/1, Cross Product5/1, Matrix Concatenate2/1

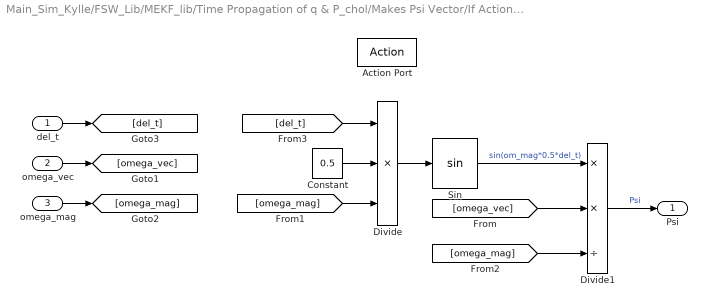
== system Main_Sim_Kylle/FSW_Lib/MEKF_lib/Time Propagation of q & P_chol/Makes Psi Vector/If Action Subsystem ==
  del_t : Inport
  omega_vec : Inport  Port=2
  omega_mag : Inport  Port=3
  Action Port : ActionPort  ActionType=else
  Constant : Constant  Value=0.5
  Divide : Product  Inputs=***
  Divide1 : Product  Inputs=**/
  Sin : Trigonometry
  Psi : Outport
  wires:
  [del_t] -> Divide/1
  del_t/1 -> [del_t]
  [omega_mag] -> Divide1/3
  [omega_mag] -> Divide/3
  omega_mag/1 -> [omega_mag]
  [omega_vec] -> Divide1/2
  omega_vec/1 -> [omega_vec]
  Sin/1 -> Divide1/1  "sin(om_mag*0.5*del_t)"
  Divide/1 -> Sin/1
  Constant/1 -> Divide/2
  Divide1/1 -> Psi/1  "Psi"

== system Main_Sim_Kylle/FSW_Lib/MEKF_lib/Time Propagation of q & P_chol/Makes Psi Vector/If Action Subsystem1 ==
  Action Port : ActionPort  ActionType=then
  Constant : Constant  Value=0
  Constant1 : Constant  Value=0
  Constant2 : Constant  Value=0
  Mux : Mux  Inputs=3
  Psi_zero : Outport
  wires:
  Mux/1 -> Psi_zero/1
  Constant2/1 -> Mux/3
  Constant1/1 -> Mux/2
  Constant/1 -> Mux/1

== matlab function Main_Sim_Kylle/satelliteDynamics_lib/quat_propagation/MATLAB Function ==
  data: w input; Omega output
function Omega = skew_sym(w)
%#codegen

    w_skew = ...
        [0 w(3) -w(2);
        -w(3) 0 w(1);
        w(2) -w(1) 0];

    Omega = ...
        [0 -w';
        w w_skew];

== matlab function Main_Sim_Kylle/FSW_Lib/MEKF_lib/Choose MEKF or Propagation/Decides if Angle Between Measurements < 2.5 deg/MATLAB Function ==
  data: u input; y output
function y = fcn(u)
%#codegen
if abs(u) <=  cosd(2.5)
    y = 1;
else
y = 0;
end

== matlab function Main_Sim_Kylle/FSW_Lib/MEKF_lib/Triad Estimator/Decides if Angle Between Measurements < 2.5 deg/MATLAB Function ==
  data: u input; y output
function y = fcn(u)
%#codegen
if abs(u) <=  cosd(2.5)
    y = 1;
else
y = 0;
end
